simulink model "sm_quadcopter"  (R2022a)
settings: Solver=ode23  StartTime=0.0  StopTime=25  FixedStep=Ts  MaxStep=0.001  RelTol=1e-3  AbsTol=1e-3
model workspace (MATLAB code in the model file):
  | load('xy_data_membrane.mat');
undefined symbols (not defined in the file or in its folder): infPlane, kd_altitude, kd_attitude, kd_position, ki_altitude, ki_attitude, kp_altitude, kp_attitude, kp_position, propeller, targetX, targetY, targetZ, timespot, waypoints, X, x0, xrot, Y, y0, yrot, Z, z0, zrot
libraries: sm_lib x101, fl_lib x40, nesl_utility x36, slpidlib x4
(part 4 of 4)

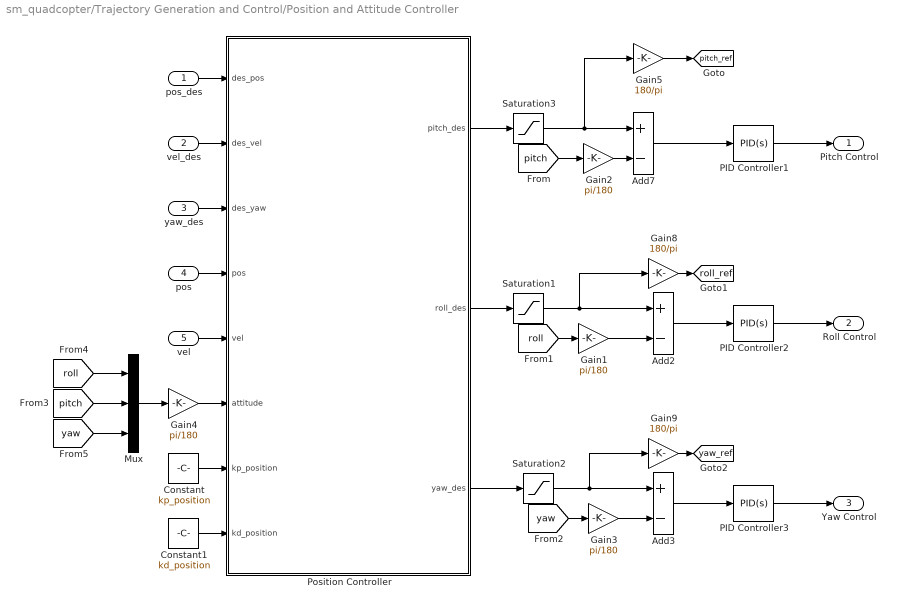
== system sm_quadcopter/Trajectory Generation and Control/Position and Attitude Controller ==
  pos_des : Inport
  vel_des : Inport  Port=2
  yaw_des : Inport  Port=3
  pos : Inport  Port=4
  vel : Inport  Port=5
  Add2 : Sum  Inputs=+-
  Add3 : Sum  Inputs=+-
  Add7 : Sum  Inputs=+-
  Constant : Constant  Value=kp_position
  Constant1 : Constant  Value=kd_position
  Gain{1..4} (4 alike) : Gain  Gain=pi/180
  Gain5 : Gain  Gain=180/pi
  Gain8 : Gain  Gain=180/pi
  Gain9 : Gain  Gain=180/pi
  Mux : Mux  Inputs=3
  PID Controller1 : slpidlib/PID Controller  Controller=PID  Form=Parallel  TimeDomain=Continuous-time  UseExternalTs=off  SampleTime=-1  IntegratorMethod=Forward Euler  FilterMethod=Forward Euler  ControllerParametersSource=internal  P=kp_attitude  I=ki_attitude  UseKiTs=off  D=kd_attitude  N=100  UseFilter=on  TunerSelectOption=Transfer Function Based (PID Tuner App)  InitialConditionSource=internal  InitialConditionForIntegrator=0  InitialConditionForFilter=0  DifferentiatorICPrevScaledInput=0  ExternalReset=none  TrackingMode=off  Kt=1  LimitOutput=on  SatLimitsSource=internal  UpperSaturationLimit=50  LowerSaturationLimit=-50  LinearizeAsGain=on  AntiWindupMode=none  Kb=1  POutMin=[]  POutMax=[]  IOutMin=[]  IOutMax=[]  DOutMin=[]  DOutMax=[]  NOutMin=[]  NOutMax=[]  SumOutMin=[]  SumOutMax=[]  SaturationOutMin=[]  SaturationOutMax=[]  PParamMin=[]  PParamMax=[]  IParamMin=[]  IParamMax=[]  DParamMin=[]  DParamMax=[]  NParamMin=[]  NParamMax=[]  KbParamMin=[]  KbParamMax=[]  KtParamMin=[]  KtParamMax=[]  KbOutMin=[]  KbOutMax=[]  KtOutMin=[]  KtOutMax=[]  IntegratorOutMin=[]  IntegratorOutMax=[]  FilterOutMin=[]  FilterOutMax=[]  SumI1OutMin=[]  SumI1OutMax=[]  SumI2OutMin=[]  SumI2OutMax=[]  SumI3OutMin=[]  SumI3OutMax=[]  SumI4OutMin=[]  SumI4OutMax=[]  SumDOutMin=[]  SumDOutMax=[]  DifferentiatorOutMin=[]  DifferentiatorOutMax=[]  FilterDiffOutCoefMin=[]  FilterDiffOutCoefMax=[]  ReciprocalOutMin=[]  ReciprocalOutMax=[]  SumDenOutMin=[]  SumDenOutMax=[]  SumNumOutMin=[]  SumNumOutMax=[]  DivideOutMin=[]  DivideOutMax=[]  UdiffTsProdOutMin=[]  UdiffTsProdOutMax=[]  NTsProdOutMin=[]  NTsProdOutMax=[]  UintegralTsProdOutMin=[]  UintegralTsProdOutMax=[]  UngainTsProdOutMin=[]  UngainTsProdOutMax=[]  IntegratorContinuousStateAttributes=''  IntegratorStateMustResolveToSignalObject=off  IntegratorRTWStateStorageClass=Auto  FilterContinuousStateAttributes=''  FilterStateMustResolveToSignalObject=off  FilterRTWStateStorageClass=Auto  ParallelPVariant=InternalParameters  IdealPVariant=Disabled  IVariant=InternalParameters  DVariant=InternalParameters  IntegratorVariant=Continuous  SatVariant=Enabled  AWVariant=Passthrough  PCopyVariant=Disabled  TRVariant=Disabled  FdbkBlocksVariant=Forward  IdealPFdbkVariant=Disabled  SatFdbkVariant=Disabled  DerivativeFilterVariant=ContFilter  NVariant=InternalParameters  NCopyVariant=Disabled  FilterICVariant=InternalICsFilter  IntegratorICVariant=InternalICs  ExternalResetVariant=Disabled  TRSumVariant=Passthrough  SumFdbkVariant=Disabled  SumVariant=Sum_PID  TsampFilterVariant=InternalTs  TsampNgainVariant=Passthrough  TsampIntegralVariant=Passthrough  ExternalSaturationOutDataTypeStr=Inherit: Same as second input  aMode=0
  PID Controller2 : slpidlib/PID Controller  Controller=PID  Form=Parallel  TimeDomain=Continuous-time  UseExternalTs=off  SampleTime=-1  IntegratorMethod=Forward Euler  FilterMethod=Forward Euler  ControllerParametersSource=internal  P=kp_attitude  I=ki_attitude  UseKiTs=off  D=kd_attitude  N=100  UseFilter=on  TunerSelectOption=Transfer Function Based (PID Tuner App)  InitialConditionSource=internal  InitialConditionForIntegrator=0  InitialConditionForFilter=0  DifferentiatorICPrevScaledInput=0  ExternalReset=none  TrackingMode=off  Kt=1  LimitOutput=on  SatLimitsSource=internal  UpperSaturationLimit=50  LowerSaturationLimit=-50  LinearizeAsGain=on  AntiWindupMode=none  Kb=1  POutMin=[]  POutMax=[]  IOutMin=[]  IOutMax=[]  DOutMin=[]  DOutMax=[]  NOutMin=[]  NOutMax=[]  SumOutMin=[]  SumOutMax=[]  SaturationOutMin=[]  SaturationOutMax=[]  PParamMin=[]  PParamMax=[]  IParamMin=[]  IParamMax=[]  DParamMin=[]  DParamMax=[]  NParamMin=[]  NParamMax=[]  KbParamMin=[]  KbParamMax=[]  KtParamMin=[]  KtParamMax=[]  KbOutMin=[]  KbOutMax=[]  KtOutMin=[]  KtOutMax=[]  IntegratorOutMin=[]  IntegratorOutMax=[]  FilterOutMin=[]  FilterOutMax=[]  SumI1OutMin=[]  SumI1OutMax=[]  SumI2OutMin=[]  SumI2OutMax=[]  SumI3OutMin=[]  SumI3OutMax=[]  SumI4OutMin=[]  SumI4OutMax=[]  SumDOutMin=[]  SumDOutMax=[]  DifferentiatorOutMin=[]  DifferentiatorOutMax=[]  FilterDiffOutCoefMin=[]  FilterDiffOutCoefMax=[]  ReciprocalOutMin=[]  ReciprocalOutMax=[]  SumDenOutMin=[]  SumDenOutMax=[]  SumNumOutMin=[]  SumNumOutMax=[]  DivideOutMin=[]  DivideOutMax=[]  UdiffTsProdOutMin=[]  UdiffTsProdOutMax=[]  NTsProdOutMin=[]  NTsProdOutMax=[]  UintegralTsProdOutMin=[]  UintegralTsProdOutMax=[]  UngainTsProdOutMin=[]  UngainTsProdOutMax=[]  IntegratorContinuousStateAttributes=''  IntegratorStateMustResolveToSignalObject=off  IntegratorRTWStateStorageClass=Auto  FilterContinuousStateAttributes=''  FilterStateMustResolveToSignalObject=off  FilterRTWStateStorageClass=Auto  ParallelPVariant=InternalParameters  IdealPVariant=Disabled  IVariant=InternalParameters  DVariant=InternalParameters  IntegratorVariant=Continuous  SatVariant=Enabled  AWVariant=Passthrough  PCopyVariant=Disabled  TRVariant=Disabled  FdbkBlocksVariant=Forward  IdealPFdbkVariant=Disabled  SatFdbkVariant=Disabled  DerivativeFilterVariant=ContFilter  NVariant=InternalParameters  NCopyVariant=Disabled  FilterICVariant=InternalICsFilter  IntegratorICVariant=InternalICs  ExternalResetVariant=Disabled  TRSumVariant=Passthrough  SumFdbkVariant=Disabled  SumVariant=Sum_PID  TsampFilterVariant=InternalTs  TsampNgainVariant=Passthrough  TsampIntegralVariant=Passthrough  ExternalSaturationOutDataTypeStr=Inherit: Same as second input  aMode=0
  PID Controller3 : slpidlib/PID Controller  Controller=PID  Form=Parallel  TimeDomain=Continuous-time  UseExternalTs=off  SampleTime=-1  IntegratorMethod=Forward Euler  FilterMethod=Forward Euler  ControllerParametersSource=internal  P=kp_attitude  I=ki_attitude  UseKiTs=off  D=kd_attitude  N=100  UseFilter=on  TunerSelectOption=Transfer Function Based (PID Tuner App)  InitialConditionSource=internal  InitialConditionForIntegrator=0  InitialConditionForFilter=0  DifferentiatorICPrevScaledInput=0  ExternalReset=none  TrackingMode=off  Kt=1  LimitOutput=on  SatLimitsSource=internal  UpperSaturationLimit=50  LowerSaturationLimit=-50  LinearizeAsGain=on  AntiWindupMode=none  Kb=1  POutMin=[]  POutMax=[]  IOutMin=[]  IOutMax=[]  DOutMin=[]  DOutMax=[]  NOutMin=[]  NOutMax=[]  SumOutMin=[]  SumOutMax=[]  SaturationOutMin=[]  SaturationOutMax=[]  PParamMin=[]  PParamMax=[]  IParamMin=[]  IParamMax=[]  DParamMin=[]  DParamMax=[]  NParamMin=[]  NParamMax=[]  KbParamMin=[]  KbParamMax=[]  KtParamMin=[]  KtParamMax=[]  KbOutMin=[]  KbOutMax=[]  KtOutMin=[]  KtOutMax=[]  IntegratorOutMin=[]  IntegratorOutMax=[]  FilterOutMin=[]  FilterOutMax=[]  SumI1OutMin=[]  SumI1OutMax=[]  SumI2OutMin=[]  SumI2OutMax=[]  SumI3OutMin=[]  SumI3OutMax=[]  SumI4OutMin=[]  SumI4OutMax=[]  SumDOutMin=[]  SumDOutMax=[]  DifferentiatorOutMin=[]  DifferentiatorOutMax=[]  FilterDiffOutCoefMin=[]  FilterDiffOutCoefMax=[]  ReciprocalOutMin=[]  ReciprocalOutMax=[]  SumDenOutMin=[]  SumDenOutMax=[]  SumNumOutMin=[]  SumNumOutMax=[]  DivideOutMin=[]  DivideOutMax=[]  UdiffTsProdOutMin=[]  UdiffTsProdOutMax=[]  NTsProdOutMin=[]  NTsProdOutMax=[]  UintegralTsProdOutMin=[]  UintegralTsProdOutMax=[]  UngainTsProdOutMin=[]  UngainTsProdOutMax=[]  IntegratorContinuousStateAttributes=''  IntegratorStateMustResolveToSignalObject=off  IntegratorRTWStateStorageClass=Auto  FilterContinuousStateAttributes=''  FilterStateMustResolveToSignalObject=off  FilterRTWStateStorageClass=Auto  ParallelPVariant=InternalParameters  IdealPVariant=Disabled  IVariant=InternalParameters  DVariant=InternalParameters  IntegratorVariant=Continuous  SatVariant=Enabled  AWVariant=Passthrough  PCopyVariant=Disabled  TRVariant=Disabled  FdbkBlocksVariant=Forward  IdealPFdbkVariant=Disabled  SatFdbkVariant=Disabled  DerivativeFilterVariant=ContFilter  NVariant=InternalParameters  NCopyVariant=Disabled  FilterICVariant=InternalICsFilter  IntegratorICVariant=InternalICs  ExternalResetVariant=Disabled  TRSumVariant=Passthrough  SumFdbkVariant=Disabled  SumVariant=Sum_PID  TsampFilterVariant=InternalTs  TsampNgainVariant=Passthrough  TsampIntegralVariant=Passthrough  ExternalSaturationOutDataTypeStr=Inherit: Same as second input  aMode=0
  Position Controller : MATLAB Function  TreatAsAtomicUnit=on
  Saturation1 : Saturate  UpperLimit=pi/3  LowerLimit=-pi/3
  Saturation2 : Saturate  UpperLimit=pi/3  LowerLimit=-pi/3
  Saturation3 : Saturate  UpperLimit=pi/3  LowerLimit=-pi/3
  Pitch Control : Outport
  Roll Control : Outport  Port=2
  Yaw Control : Outport  Port=3
  tag scope: pitch_ref=global, roll_ref=global, yaw_ref=global
  wires:
  pos/1 -> Position Controller/4(pos)
  pos_des/1 -> Position Controller/1(des_pos)
  Position Controller/2(roll_des) -> Saturation1/1
  Saturation2/1 -> Gain9/1, Add3/1
  Position Controller/3(yaw_des) -> Saturation2/1
  yaw_des/1 -> Position Controller/3(des_yaw)
  vel/1 -> Position Controller/5(vel)
  [yaw] -> Gain3/1
  [roll] -> Gain1/1
  [pitch] -> Gain2/1
  vel_des/1 -> Position Controller/2(des_vel)
  Saturation1/1 -> Gain8/1, Add2/1
  Saturation3/1 -> Add7/1, Gain5/1
  Position Controller/1(pitch_des) -> Saturation3/1
  Mux/1 -> Gain4/1
  [roll] -> Mux/1
  [pitch] -> Mux/2
  [yaw] -> Mux/3
  Gain4/1 -> Position Controller/6(attitude)
  Gain1/1 -> Add2/2
  Gain3/1 -> Add3/2
  Gain5/1 -> [pitch_ref]
  Gain8/1 -> [roll_ref]
  Gain9/1 -> [yaw_ref]
  Gain2/1 -> Add7/2
  Add7/1 -> PID Controller1/1
  PID Controller1/1 -> Pitch Control/1
  Add2/1 -> PID Controller2/1
  PID Controller2/1 -> Roll Control/1
  Add3/1 -> PID Controller3/1
  PID Controller3/1 -> Yaw Control/1
  Constant/1 -> Position Controller/7(kp_position)
  Constant1/1 -> Position Controller/8(kd_position)

== system sm_quadcopter/Package Delivery Quadcopter/Motor Propeller 1/Propeller Thrust Calculator ==
  Air Density : fl_lib/Physical Signals/Sources/PS Constant  constant=1.225 kg/m^3
      settings: SourceProductBaseCode=PW,SS,VE
  PS Gain : fl_lib/Physical Signals/Functions/PS Gain  gain=1/60
      settings: SourceProductBaseCode=PW,SS,VE
  PS Math Function : fl_lib/Physical Signals/Functions/PS Math Function  fcn_choice=foundation.enum.math_function.pow  v=4
      settings: SourceProductBaseCode=PW,SS,VE
  PS Math Function1 : fl_lib/Physical Signals/Functions/PS Math Function  fcn_choice=foundation.enum.math_function.square  v=2
      settings: SourceProductBaseCode=PW,SS,VE
  PS Product : fl_lib/Physical Signals/Functions/PS Product
      settings: SourceProductBaseCode=PW,SS,VE
  PS Product1 : fl_lib/Physical Signals/Functions/PS Product
      settings: SourceProductBaseCode=PW,SS,VE
  PS Product2 : fl_lib/Physical Signals/Functions/PS Product
      settings: SourceProductBaseCode=PW,SS,VE
  Propeller Diameter : fl_lib/Physical Signals/Sources/PS Constant  constant=propeller.diameter m
      settings: SourceProductBaseCode=PW,SS,VE
  Ct : PMIOPort  Side=Left
  Propeller Speed : PMIOPort  Port=2  Side=Left
  Thrust : PMIOPort  Port=3  Side=Right
  connections:
  PS Math Function/LConn1 -- Propeller Diameter/RConn1
  PS Math Function1/RConn1 -- PS Product1/LConn1
  Air Density/RConn1 -- PS Product1/LConn2
  PS Product1/RConn1 -- PS Product2/LConn2
  PS Gain/RConn1 -- PS Math Function1/LConn1
  PS Math Function/RConn1 -- PS Product/LConn2
  PS Product/RConn1 -- PS Product2/LConn1
  Propeller Speed/RConn1 -- PS Gain/LConn1
  Thrust/RConn1 -- PS Product2/RConn1
  PS Product/LConn1 -- Ct/RConn1

== system sm_quadcopter/Package Delivery Quadcopter/Motor Propeller 1/Thrust Coefficient Calculator ==
  m/s : Inport
  Add : Sum  Inputs=+++
  Constant : Constant  Value=0.1072
  Gain1 : Gain  Gain=-0.008716
  Gain4 : Gain  Gain=-0.001589
  Math Function : Math  Operator=square
  Simulink-PS Converter : nesl_utility/Simulink-PS Converter  PhysicalDomain=network_engine_domain  SubClassName=ps_input  LeftPortType=input  RightPortType=output  PseudoPeriodic=off  Frequencies=[]  NoiseDistribution=none  NoiseParameters=[]  Unit=1/(rev)^2  AffineConversion=off  FilteringAndDerivatives=provide  SimscapeFilterOrder=1  InputFilterTimeConstant=0.001  UdotUserProvided=0
      settings: SourceProductBaseCode=SS,PW,VE
  Ct : PMIOPort  Side=Right
  wires:
  Constant/1 -> Add/3
  Gain4/1 -> Add/1
  Add/1 -> Simulink-PS Converter/1
  m/s/1 -> Gain1/1, Math Function/1
  Math Function/1 -> Gain4/1
  Gain1/1 -> Add/2
  connections:
  Simulink-PS Converter/RConn1 -- Ct/RConn1

== system sm_quadcopter/Package Delivery Quadcopter/Motor Propeller 2/Propeller Thrust Calculator ==
  Air Density : fl_lib/Physical Signals/Sources/PS Constant  constant=1.225 kg/m^3
      settings: SourceProductBaseCode=PW,SS,VE
  PS Gain : fl_lib/Physical Signals/Functions/PS Gain  gain=1/60
      settings: SourceProductBaseCode=PW,SS,VE
  PS Math Function : fl_lib/Physical Signals/Functions/PS Math Function  fcn_choice=foundation.enum.math_function.pow  v=4
      settings: SourceProductBaseCode=PW,SS,VE
  PS Math Function1 : fl_lib/Physical Signals/Functions/PS Math Function  fcn_choice=foundation.enum.math_function.square  v=2
      settings: SourceProductBaseCode=PW,SS,VE
  PS Product : fl_lib/Physical Signals/Functions/PS Product
      settings: SourceProductBaseCode=PW,SS,VE
  PS Product1 : fl_lib/Physical Signals/Functions/PS Product
      settings: SourceProductBaseCode=PW,SS,VE
  PS Product2 : fl_lib/Physical Signals/Functions/PS Product
      settings: SourceProductBaseCode=PW,SS,VE
  Propeller Diameter : fl_lib/Physical Signals/Sources/PS Constant  constant=propeller.diameter m
      settings: SourceProductBaseCode=PW,SS,VE
  Ct : PMIOPort  Side=Left
  Propeller Speed : PMIOPort  Port=2  Side=Left
  Thrust : PMIOPort  Port=3  Side=Right
  connections:
  PS Math Function/LConn1 -- Propeller Diameter/RConn1
  PS Math Function1/RConn1 -- PS Product1/LConn1
  Air Density/RConn1 -- PS Product1/LConn2
  PS Product1/RConn1 -- PS Product2/LConn2
  PS Gain/RConn1 -- PS Math Function1/LConn1
  PS Math Function/RConn1 -- PS Product/LConn2
  PS Product/RConn1 -- PS Product2/LConn1
  Propeller Speed/RConn1 -- PS Gain/LConn1
  Thrust/RConn1 -- PS Product2/RConn1
  PS Product/LConn1 -- Ct/RConn1

== system sm_quadcopter/Package Delivery Quadcopter/Motor Propeller 2/Thrust Coefficient Calculator ==
  m/s : Inport
  Add : Sum  Inputs=+++
  Constant : Constant  Value=0.1072
  Gain1 : Gain  Gain=-0.008716
  Gain4 : Gain  Gain=-0.001589
  Math Function : Math  Operator=square
  Simulink-PS Converter : nesl_utility/Simulink-PS Converter  PhysicalDomain=network_engine_domain  SubClassName=ps_input  LeftPortType=input  RightPortType=output  PseudoPeriodic=off  Frequencies=[]  NoiseDistribution=none  NoiseParameters=[]  Unit=1/(rev^2)  AffineConversion=off  FilteringAndDerivatives=provide  SimscapeFilterOrder=1  InputFilterTimeConstant=0.001  UdotUserProvided=0
      settings: SourceProductBaseCode=SS,PW,VE
  Ct : PMIOPort  Side=Right
  wires:
  Math Function/1 -> Gain4/1
  m/s/1 -> Gain1/1, Math Function/1
  Add/1 -> Simulink-PS Converter/1
  Gain4/1 -> Add/1
  Gain1/1 -> Add/2
  Constant/1 -> Add/3
  connections:
  Simulink-PS Converter/RConn1 -- Ct/RConn1

== system sm_quadcopter/Package Delivery Quadcopter/Motor Propeller 3 /Propeller Thrust Calculator ==
  Air Density : fl_lib/Physical Signals/Sources/PS Constant  constant=1.225 kg/m^3
      settings: SourceProductBaseCode=PW,SS,VE
  PS Gain : fl_lib/Physical Signals/Functions/PS Gain  gain=1/60
      settings: SourceProductBaseCode=PW,SS,VE
  PS Math Function : fl_lib/Physical Signals/Functions/PS Math Function  fcn_choice=foundation.enum.math_function.pow  v=4
      settings: SourceProductBaseCode=PW,SS,VE
  PS Math Function1 : fl_lib/Physical Signals/Functions/PS Math Function  fcn_choice=foundation.enum.math_function.square  v=2
      settings: SourceProductBaseCode=PW,SS,VE
  PS Product : fl_lib/Physical Signals/Functions/PS Product
      settings: SourceProductBaseCode=PW,SS,VE
  PS Product1 : fl_lib/Physical Signals/Functions/PS Product
      settings: SourceProductBaseCode=PW,SS,VE
  PS Product2 : fl_lib/Physical Signals/Functions/PS Product
      settings: SourceProductBaseCode=PW,SS,VE
  Propeller Diameter : fl_lib/Physical Signals/Sources/PS Constant  constant=propeller.diameter m
      settings: SourceProductBaseCode=PW,SS,VE
  Ct : PMIOPort  Side=Left
  Propeller Speed : PMIOPort  Port=2  Side=Left
  Thrust : PMIOPort  Port=3  Side=Right
  connections:
  PS Math Function/LConn1 -- Propeller Diameter/RConn1
  PS Math Function1/RConn1 -- PS Product1/LConn1
  Air Density/RConn1 -- PS Product1/LConn2
  PS Product1/RConn1 -- PS Product2/LConn2
  PS Math Function/RConn1 -- PS Product/LConn2
  PS Product/RConn1 -- PS Product2/LConn1
  PS Math Function1/LConn1 -- PS Gain/RConn1
  Propeller Speed/RConn1 -- PS Gain/LConn1
  Thrust/RConn1 -- PS Product2/RConn1
  PS Product/LConn1 -- Ct/RConn1

== system sm_quadcopter/Package Delivery Quadcopter/Motor Propeller 3 /Thrust Coefficient Calculator ==
  m/s : Inport
  Add : Sum  Inputs=+++
  Constant : Constant  Value=0.1072
  Gain1 : Gain  Gain=-0.008716
  Gain4 : Gain  Gain=-0.001589
  Math Function : Math  Operator=square
  Simulink-PS Converter : nesl_utility/Simulink-PS Converter  PhysicalDomain=network_engine_domain  SubClassName=ps_input  LeftPortType=input  RightPortType=output  PseudoPeriodic=off  Frequencies=[]  NoiseDistribution=none  NoiseParameters=[]  Unit=1/(rev)^2  AffineConversion=off  FilteringAndDerivatives=provide  SimscapeFilterOrder=1  InputFilterTimeConstant=0.001  UdotUserProvided=0
      settings: SourceProductBaseCode=SS,PW,VE
  Ct : PMIOPort  Side=Right
  wires:
  Constant/1 -> Add/3
  Gain4/1 -> Add/1
  Add/1 -> Simulink-PS Converter/1
  m/s/1 -> Gain1/1, Math Function/1
  Math Function/1 -> Gain4/1
  Gain1/1 -> Add/2
  connections:
  Simulink-PS Converter/RConn1 -- Ct/RConn1

== system sm_quadcopter/Package Delivery Quadcopter/Motor Propeller 4/Propeller Thrust Calculator ==
  Air Density : fl_lib/Physical Signals/Sources/PS Constant  constant=1.225 kg/m^3
      settings: SourceProductBaseCode=PW,SS,VE
  PS Gain : fl_lib/Physical Signals/Functions/PS Gain  gain=1/60
      settings: SourceProductBaseCode=PW,SS,VE
  PS Math Function : fl_lib/Physical Signals/Functions/PS Math Function  fcn_choice=foundation.enum.math_function.pow  v=4
      settings: SourceProductBaseCode=PW,SS,VE
  PS Math Function1 : fl_lib/Physical Signals/Functions/PS Math Function  fcn_choice=foundation.enum.math_function.square  v=2
      settings: SourceProductBaseCode=PW,SS,VE
  PS Product : fl_lib/Physical Signals/Functions/PS Product
      settings: SourceProductBaseCode=PW,SS,VE
  PS Product1 : fl_lib/Physical Signals/Functions/PS Product
      settings: SourceProductBaseCode=PW,SS,VE
  PS Product2 : fl_lib/Physical Signals/Functions/PS Product
      settings: SourceProductBaseCode=PW,SS,VE
  Propeller Diameter : fl_lib/Physical Signals/Sources/PS Constant  constant=propeller.diameter m
      settings: SourceProductBaseCode=PW,SS,VE
  Ct : PMIOPort  Side=Left
  Propeller Speed : PMIOPort  Port=2  Side=Left
  Thrust : PMIOPort  Port=3  Side=Right
  connections:
  PS Math Function/LConn1 -- Propeller Diameter/RConn1
  PS Math Function1/RConn1 -- PS Product1/LConn1
  Air Density/RConn1 -- PS Product1/LConn2
  PS Product1/RConn1 -- PS Product2/LConn2
  PS Gain/RConn1 -- PS Math Function1/LConn1
  PS Math Function/RConn1 -- PS Product/LConn2
  PS Product/RConn1 -- PS Product2/LConn1
  Propeller Speed/RConn1 -- PS Gain/LConn1
  Thrust/RConn1 -- PS Product2/RConn1
  PS Product/LConn1 -- Ct/RConn1

== system sm_quadcopter/Package Delivery Quadcopter/Motor Propeller 4/Thrust Coefficient Calculator ==
  m/s : Inport
  Add : Sum  Inputs=+++
  Constant : Constant  Value=0.1072
  Gain1 : Gain  Gain=-0.008716
  Gain4 : Gain  Gain=-0.001589
  Math Function : Math  Operator=square
  Simulink-PS Converter : nesl_utility/Simulink-PS Converter  PhysicalDomain=network_engine_domain  SubClassName=ps_input  LeftPortType=input  RightPortType=output  PseudoPeriodic=off  Frequencies=[]  NoiseDistribution=none  NoiseParameters=[]  Unit=1/(rev)^2  AffineConversion=off  FilteringAndDerivatives=provide  SimscapeFilterOrder=1  InputFilterTimeConstant=0.001  UdotUserProvided=0
      settings: SourceProductBaseCode=SS,PW,VE
  Ct : PMIOPort  Side=Right
  wires:
  Constant/1 -> Add/3
  Gain4/1 -> Add/1
  Add/1 -> Simulink-PS Converter/1
  m/s/1 -> Gain1/1, Math Function/1
  Math Function/1 -> Gain4/1
  Gain1/1 -> Add/2
  connections:
  Simulink-PS Converter/RConn1 -- Ct/RConn1

== system sm_quadcopter/Package Delivery Quadcopter/Package/Subsystem ==
  Spatial Contact Force : sm_lib/Forces and Torques/Spatial Contact Force  SenseContactBaseRotation=off  SenseContactBaseTranslation=off  CoefficientOfDynamicFriction=0.3  CoefficientOfStaticFriction=0.5  NormalDamping=pkgGrndDamp  NormalDampingUnits=N/(m/s)  SenseContactSignal=off  NormalStiffness=pkgGrndStiff  NormalStiffnessUnits=N/m  FrictionalCriticalVelocity=1e-2  FrictionalCriticalVelocityUnits=m/s  ZeroCrossDetectContactStartAndEnd=off  SenseContactFollowerRotation=off  SenseContactFollowerTranslation=off  FrictionType=SmoothStickSlip  SenseFrictionalForceMagnitude=off  SenseNormalForceMagnitude=off  NormalForceType=SmoothSpringDamper  SenseNormalVelocity=off  SenseSeparationDistance=off  SenseTangentialVelocity=off  NormalTransitionRegionWidth=pkgGrndTransW  NormalTransitionRegionWidthUnits=m
  Spherical Solid : sm_lib/Body Elements/Spherical Solid  GraphicAmbientColor=[0.15 0.15 0.15 1.0]  BasedOnType=Density  CenterOfMass=[0 0 0]  CenterOfMassUnits=m  GraphicDiffuseColor=[0.5 0.5 0.5]  Density=1  DensityUnits=kg/m^3  DoExposeReferenceFrame=on  GraphicEmissiveColor=[0.0 0.0 0.0 1.0]  ExportEntireGeometry=on  SerializedExposedGeometries=<ExposedGeometries><ExposedGeometry><RawGeometryId>entire</RawGeometryId><ExposedGeometryId>G</ExposedGeometryId></ExposedGeometry></ExposedGeometries>  SerializedFrames=<Frames/>  MarkerShape=Sphere  MarkerSize=10  GraphicType=FromGeometry  InertiaType=CalculateFromGeometry  Mass=1  MassUnits=kg  MomentsOfInertia=[1 1 1]  MomentsOfInertiaUnits=kg*m^2  GraphicOpacity=1.0  ProductsOfInertia=[0 0 0]  ProductsOfInertiaUnits=kg*m^2  GraphicShininess=75  GraphicSpecularColor=[0.5 0.5 0.5 1.0]  SphereRadius=0.0025  SphereRadiusUnits=m  GraphicVisPropType=SimpleVisualProperties
  R : PMIOPort  Side=Right
  G : PMIOPort  Port=2  Side=Left
  connections:
  Spatial Contact Force/LConn1 -- Spherical Solid/LConn1
  Spherical Solid/RConn1 -- R/RConn1
  Spatial Contact Force/RConn1 -- G/RConn1

== system sm_quadcopter/Package Delivery Quadcopter/Package/Subsystem1 ==
  Spatial Contact Force : sm_lib/Forces and Torques/Spatial Contact Force  SenseContactBaseRotation=off  SenseContactBaseTranslation=off  CoefficientOfDynamicFriction=0.3  CoefficientOfStaticFriction=0.5  NormalDamping=pkgGrndDamp  NormalDampingUnits=N/(m/s)  SenseContactSignal=off  NormalStiffness=pkgGrndStiff  NormalStiffnessUnits=N/m  FrictionalCriticalVelocity=1e-2  FrictionalCriticalVelocityUnits=m/s  ZeroCrossDetectContactStartAndEnd=off  SenseContactFollowerRotation=off  SenseContactFollowerTranslation=off  FrictionType=SmoothStickSlip  SenseFrictionalForceMagnitude=off  SenseNormalForceMagnitude=off  NormalForceType=SmoothSpringDamper  SenseNormalVelocity=off  SenseSeparationDistance=off  SenseTangentialVelocity=off  NormalTransitionRegionWidth=pkgGrndTransW  NormalTransitionRegionWidthUnits=m
  Spherical Solid : sm_lib/Body Elements/Spherical Solid  GraphicAmbientColor=[0.15 0.15 0.15 1.0]  BasedOnType=Density  CenterOfMass=[0 0 0]  CenterOfMassUnits=m  GraphicDiffuseColor=[0.5 0.5 0.5]  Density=1  DensityUnits=kg/m^3  DoExposeReferenceFrame=on  GraphicEmissiveColor=[0.0 0.0 0.0 1.0]  ExportEntireGeometry=on  SerializedExposedGeometries=<ExposedGeometries><ExposedGeometry><RawGeometryId>entire</RawGeometryId><ExposedGeometryId>G</ExposedGeometryId></ExposedGeometry></ExposedGeometries>  SerializedFrames=<Frames/>  MarkerShape=Sphere  MarkerSize=10  GraphicType=FromGeometry  InertiaType=CalculateFromGeometry  Mass=1  MassUnits=kg  MomentsOfInertia=[1 1 1]  MomentsOfInertiaUnits=kg*m^2  GraphicOpacity=1.0  ProductsOfInertia=[0 0 0]  ProductsOfInertiaUnits=kg*m^2  GraphicShininess=75  GraphicSpecularColor=[0.5 0.5 0.5 1.0]  SphereRadius=0.0025  SphereRadiusUnits=m  GraphicVisPropType=SimpleVisualProperties
  R : PMIOPort  Side=Right
  G : PMIOPort  Port=2  Side=Left
  connections:
  Spatial Contact Force/RConn1 -- G/RConn1
  Spherical Solid/RConn1 -- R/RConn1
  Spatial Contact Force/LConn1 -- Spherical Solid/LConn1

== system sm_quadcopter/Package Delivery Quadcopter/Package/Subsystem2 ==
  Spatial Contact Force : sm_lib/Forces and Torques/Spatial Contact Force  SenseContactBaseRotation=off  SenseContactBaseTranslation=off  CoefficientOfDynamicFriction=0.3  CoefficientOfStaticFriction=0.5  NormalDamping=pkgGrndDamp  NormalDampingUnits=N/(m/s)  SenseContactSignal=off  NormalStiffness=pkgGrndStiff  NormalStiffnessUnits=N/m  FrictionalCriticalVelocity=1e-2  FrictionalCriticalVelocityUnits=m/s  ZeroCrossDetectContactStartAndEnd=off  SenseContactFollowerRotation=off  SenseContactFollowerTranslation=off  FrictionType=SmoothStickSlip  SenseFrictionalForceMagnitude=off  SenseNormalForceMagnitude=off  NormalForceType=SmoothSpringDamper  SenseNormalVelocity=off  SenseSeparationDistance=off  SenseTangentialVelocity=off  NormalTransitionRegionWidth=pkgGrndTransW  NormalTransitionRegionWidthUnits=m
  Spherical Solid : sm_lib/Body Elements/Spherical Solid  GraphicAmbientColor=[0.15 0.15 0.15 1.0]  BasedOnType=Density  CenterOfMass=[0 0 0]  CenterOfMassUnits=m  GraphicDiffuseColor=[0.5 0.5 0.5]  Density=1  DensityUnits=kg/m^3  DoExposeReferenceFrame=on  GraphicEmissiveColor=[0.0 0.0 0.0 1.0]  ExportEntireGeometry=on  SerializedExposedGeometries=<ExposedGeometries><ExposedGeometry><RawGeometryId>entire</RawGeometryId><ExposedGeometryId>G</ExposedGeometryId></ExposedGeometry></ExposedGeometries>  SerializedFrames=<Frames/>  MarkerShape=Sphere  MarkerSize=10  GraphicType=FromGeometry  InertiaType=CalculateFromGeometry  Mass=1  MassUnits=kg  MomentsOfInertia=[1 1 1]  MomentsOfInertiaUnits=kg*m^2  GraphicOpacity=1.0  ProductsOfInertia=[0 0 0]  ProductsOfInertiaUnits=kg*m^2  GraphicShininess=75  GraphicSpecularColor=[0.5 0.5 0.5 1.0]  SphereRadius=0.0025  SphereRadiusUnits=m  GraphicVisPropType=SimpleVisualProperties
  R : PMIOPort  Side=Right
  G : PMIOPort  Port=2  Side=Left
  connections:
  Spatial Contact Force/LConn1 -- Spherical Solid/LConn1
  Spherical Solid/RConn1 -- R/RConn1
  Spatial Contact Force/RConn1 -- G/RConn1

== system sm_quadcopter/Package Delivery Quadcopter/Package/Subsystem3 ==
  Spatial Contact Force : sm_lib/Forces and Torques/Spatial Contact Force  SenseContactBaseRotation=off  SenseContactBaseTranslation=off  CoefficientOfDynamicFriction=0.3  CoefficientOfStaticFriction=0.5  NormalDamping=pkgGrndDamp  NormalDampingUnits=N/(m/s)  SenseContactSignal=off  NormalStiffness=pkgGrndStiff  NormalStiffnessUnits=N/m  FrictionalCriticalVelocity=1e-2  FrictionalCriticalVelocityUnits=m/s  ZeroCrossDetectContactStartAndEnd=off  SenseContactFollowerRotation=off  SenseContactFollowerTranslation=off  FrictionType=SmoothStickSlip  SenseFrictionalForceMagnitude=off  SenseNormalForceMagnitude=off  NormalForceType=SmoothSpringDamper  SenseNormalVelocity=off  SenseSeparationDistance=off  SenseTangentialVelocity=off  NormalTransitionRegionWidth=pkgGrndTransW  NormalTransitionRegionWidthUnits=m
  Spherical Solid : sm_lib/Body Elements/Spherical Solid  GraphicAmbientColor=[0.15 0.15 0.15 1.0]  BasedOnType=Density  CenterOfMass=[0 0 0]  CenterOfMassUnits=m  GraphicDiffuseColor=[0.5 0.5 0.5]  Density=1  DensityUnits=kg/m^3  DoExposeReferenceFrame=on  GraphicEmissiveColor=[0.0 0.0 0.0 1.0]  ExportEntireGeometry=on  SerializedExposedGeometries=<ExposedGeometries><ExposedGeometry><RawGeometryId>entire</RawGeometryId><ExposedGeometryId>G</ExposedGeometryId></ExposedGeometry></ExposedGeometries>  SerializedFrames=<Frames/>  MarkerShape=Sphere  MarkerSize=10  GraphicType=FromGeometry  InertiaType=CalculateFromGeometry  Mass=1  MassUnits=kg  MomentsOfInertia=[1 1 1]  MomentsOfInertiaUnits=kg*m^2  GraphicOpacity=1.0  ProductsOfInertia=[0 0 0]  ProductsOfInertiaUnits=kg*m^2  GraphicShininess=75  GraphicSpecularColor=[0.5 0.5 0.5 1.0]  SphereRadius=0.0025  SphereRadiusUnits=m  GraphicVisPropType=SimpleVisualProperties
  R : PMIOPort  Side=Right
  G : PMIOPort  Port=2  Side=Left
  connections:
  Spatial Contact Force/RConn1 -- G/RConn1
  Spherical Solid/RConn1 -- R/RConn1
  Spatial Contact Force/LConn1 -- Spherical Solid/LConn1

== system sm_quadcopter/Package Delivery Quadcopter/Package/Subsystem4 ==
  Spatial Contact Force : sm_lib/Forces and Torques/Spatial Contact Force  SenseContactBaseRotation=off  SenseContactBaseTranslation=off  CoefficientOfDynamicFriction=0.3  CoefficientOfStaticFriction=0.5  NormalDamping=pkgGrndDamp  NormalDampingUnits=N/(m/s)  SenseContactSignal=off  NormalStiffness=pkgGrndStiff  NormalStiffnessUnits=N/m  FrictionalCriticalVelocity=1e-2  FrictionalCriticalVelocityUnits=m/s  ZeroCrossDetectContactStartAndEnd=off  SenseContactFollowerRotation=off  SenseContactFollowerTranslation=off  FrictionType=SmoothStickSlip  SenseFrictionalForceMagnitude=off  SenseNormalForceMagnitude=off  NormalForceType=SmoothSpringDamper  SenseNormalVelocity=off  SenseSeparationDistance=off  SenseTangentialVelocity=off  NormalTransitionRegionWidth=pkgGrndTransW  NormalTransitionRegionWidthUnits=m
  Spherical Solid : sm_lib/Body Elements/Spherical Solid  GraphicAmbientColor=[0.15 0.15 0.15 1.0]  BasedOnType=Density  CenterOfMass=[0 0 0]  CenterOfMassUnits=m  GraphicDiffuseColor=[0.5 0.5 0.5]  Density=1  DensityUnits=kg/m^3  DoExposeReferenceFrame=on  GraphicEmissiveColor=[0.0 0.0 0.0 1.0]  ExportEntireGeometry=on  SerializedExposedGeometries=<ExposedGeometries><ExposedGeometry><RawGeometryId>entire</RawGeometryId><ExposedGeometryId>G</ExposedGeometryId></ExposedGeometry></ExposedGeometries>  SerializedFrames=<Frames/>  MarkerShape=Sphere  MarkerSize=10  GraphicType=FromGeometry  InertiaType=CalculateFromGeometry  Mass=1  MassUnits=kg  MomentsOfInertia=[1 1 1]  MomentsOfInertiaUnits=kg*m^2  GraphicOpacity=1.0  ProductsOfInertia=[0 0 0]  ProductsOfInertiaUnits=kg*m^2  GraphicShininess=75  GraphicSpecularColor=[0.5 0.5 0.5 1.0]  SphereRadius=0.0025  SphereRadiusUnits=m  GraphicVisPropType=SimpleVisualProperties
  R : PMIOPort  Side=Right
  G : PMIOPort  Port=2  Side=Left
  connections:
  Spatial Contact Force/LConn1 -- Spherical Solid/LConn1
  Spherical Solid/RConn1 -- R/RConn1
  Spatial Contact Force/RConn1 -- G/RConn1

== system sm_quadcopter/Package Delivery Quadcopter/Package/Subsystem5 ==
  Spatial Contact Force : sm_lib/Forces and Torques/Spatial Contact Force  SenseContactBaseRotation=off  SenseContactBaseTranslation=off  CoefficientOfDynamicFriction=0.3  CoefficientOfStaticFriction=0.5  NormalDamping=pkgGrndDamp  NormalDampingUnits=N/(m/s)  SenseContactSignal=off  NormalStiffness=pkgGrndStiff  NormalStiffnessUnits=N/m  FrictionalCriticalVelocity=1e-2  FrictionalCriticalVelocityUnits=m/s  ZeroCrossDetectContactStartAndEnd=off  SenseContactFollowerRotation=off  SenseContactFollowerTranslation=off  FrictionType=SmoothStickSlip  SenseFrictionalForceMagnitude=off  SenseNormalForceMagnitude=off  NormalForceType=SmoothSpringDamper  SenseNormalVelocity=off  SenseSeparationDistance=off  SenseTangentialVelocity=off  NormalTransitionRegionWidth=pkgGrndTransW  NormalTransitionRegionWidthUnits=m
  Spherical Solid : sm_lib/Body Elements/Spherical Solid  GraphicAmbientColor=[0.15 0.15 0.15 1.0]  BasedOnType=Density  CenterOfMass=[0 0 0]  CenterOfMassUnits=m  GraphicDiffuseColor=[0.5 0.5 0.5]  Density=1  DensityUnits=kg/m^3  DoExposeReferenceFrame=on  GraphicEmissiveColor=[0.0 0.0 0.0 1.0]  ExportEntireGeometry=on  SerializedExposedGeometries=<ExposedGeometries><ExposedGeometry><RawGeometryId>entire</RawGeometryId><ExposedGeometryId>G</ExposedGeometryId></ExposedGeometry></ExposedGeometries>  SerializedFrames=<Frames/>  MarkerShape=Sphere  MarkerSize=10  GraphicType=FromGeometry  InertiaType=CalculateFromGeometry  Mass=1  MassUnits=kg  MomentsOfInertia=[1 1 1]  MomentsOfInertiaUnits=kg*m^2  GraphicOpacity=1.0  ProductsOfInertia=[0 0 0]  ProductsOfInertiaUnits=kg*m^2  GraphicShininess=75  GraphicSpecularColor=[0.5 0.5 0.5 1.0]  SphereRadius=0.0025  SphereRadiusUnits=m  GraphicVisPropType=SimpleVisualProperties
  R : PMIOPort  Side=Right
  G : PMIOPort  Port=2  Side=Left
  connections:
  Spatial Contact Force/RConn1 -- G/RConn1
  Spherical Solid/RConn1 -- R/RConn1
  Spatial Contact Force/LConn1 -- Spherical Solid/LConn1

== system sm_quadcopter/Package Delivery Quadcopter/Package/Subsystem6 ==
  Spatial Contact Force : sm_lib/Forces and Torques/Spatial Contact Force  SenseContactBaseRotation=off  SenseContactBaseTranslation=off  CoefficientOfDynamicFriction=0.3  CoefficientOfStaticFriction=0.5  NormalDamping=pkgGrndDamp  NormalDampingUnits=N/(m/s)  SenseContactSignal=off  NormalStiffness=pkgGrndStiff  NormalStiffnessUnits=N/m  FrictionalCriticalVelocity=1e-2  FrictionalCriticalVelocityUnits=m/s  ZeroCrossDetectContactStartAndEnd=off  SenseContactFollowerRotation=off  SenseContactFollowerTranslation=off  FrictionType=SmoothStickSlip  SenseFrictionalForceMagnitude=off  SenseNormalForceMagnitude=off  NormalForceType=SmoothSpringDamper  SenseNormalVelocity=off  SenseSeparationDistance=off  SenseTangentialVelocity=off  NormalTransitionRegionWidth=pkgGrndTransW  NormalTransitionRegionWidthUnits=m
  Spherical Solid : sm_lib/Body Elements/Spherical Solid  GraphicAmbientColor=[0.15 0.15 0.15 1.0]  BasedOnType=Density  CenterOfMass=[0 0 0]  CenterOfMassUnits=m  GraphicDiffuseColor=[0.5 0.5 0.5]  Density=1  DensityUnits=kg/m^3  DoExposeReferenceFrame=on  GraphicEmissiveColor=[0.0 0.0 0.0 1.0]  ExportEntireGeometry=on  SerializedExposedGeometries=<ExposedGeometries><ExposedGeometry><RawGeometryId>entire</RawGeometryId><ExposedGeometryId>G</ExposedGeometryId></ExposedGeometry></ExposedGeometries>  SerializedFrames=<Frames/>  MarkerShape=Sphere  MarkerSize=10  GraphicType=FromGeometry  InertiaType=CalculateFromGeometry  Mass=1  MassUnits=kg  MomentsOfInertia=[1 1 1]  MomentsOfInertiaUnits=kg*m^2  GraphicOpacity=1.0  ProductsOfInertia=[0 0 0]  ProductsOfInertiaUnits=kg*m^2  GraphicShininess=75  GraphicSpecularColor=[0.5 0.5 0.5 1.0]  SphereRadius=0.0025  SphereRadiusUnits=m  GraphicVisPropType=SimpleVisualProperties
  R : PMIOPort  Side=Right
  G : PMIOPort  Port=2  Side=Left
  connections:
  Spatial Contact Force/LConn1 -- Spherical Solid/LConn1
  Spherical Solid/RConn1 -- R/RConn1
  Spatial Contact Force/RConn1 -- G/RConn1

== system sm_quadcopter/Package Delivery Quadcopter/Package/Subsystem7 ==
  Spatial Contact Force : sm_lib/Forces and Torques/Spatial Contact Force  SenseContactBaseRotation=off  SenseContactBaseTranslation=off  CoefficientOfDynamicFriction=0.3  CoefficientOfStaticFriction=0.5  NormalDamping=pkgGrndDamp  NormalDampingUnits=N/(m/s)  SenseContactSignal=off  NormalStiffness=pkgGrndStiff  NormalStiffnessUnits=N/m  FrictionalCriticalVelocity=1e-2  FrictionalCriticalVelocityUnits=m/s  ZeroCrossDetectContactStartAndEnd=off  SenseContactFollowerRotation=off  SenseContactFollowerTranslation=off  FrictionType=SmoothStickSlip  SenseFrictionalForceMagnitude=off  SenseNormalForceMagnitude=off  NormalForceType=SmoothSpringDamper  SenseNormalVelocity=off  SenseSeparationDistance=off  SenseTangentialVelocity=off  NormalTransitionRegionWidth=pkgGrndTransW  NormalTransitionRegionWidthUnits=m
  Spherical Solid : sm_lib/Body Elements/Spherical Solid  GraphicAmbientColor=[0.15 0.15 0.15 1.0]  BasedOnType=Density  CenterOfMass=[0 0 0]  CenterOfMassUnits=m  GraphicDiffuseColor=[0.5 0.5 0.5]  Density=1  DensityUnits=kg/m^3  DoExposeReferenceFrame=on  GraphicEmissiveColor=[0.0 0.0 0.0 1.0]  ExportEntireGeometry=on  SerializedExposedGeometries=<ExposedGeometries><ExposedGeometry><RawGeometryId>entire</RawGeometryId><ExposedGeometryId>G</ExposedGeometryId></ExposedGeometry></ExposedGeometries>  SerializedFrames=<Frames/>  MarkerShape=Sphere  MarkerSize=10  GraphicType=FromGeometry  InertiaType=CalculateFromGeometry  Mass=1  MassUnits=kg  MomentsOfInertia=[1 1 1]  MomentsOfInertiaUnits=kg*m^2  GraphicOpacity=1.0  ProductsOfInertia=[0 0 0]  ProductsOfInertiaUnits=kg*m^2  GraphicShininess=75  GraphicSpecularColor=[0.5 0.5 0.5 1.0]  SphereRadius=0.0025  SphereRadiusUnits=m  GraphicVisPropType=SimpleVisualProperties
  R : PMIOPort  Side=Right
  G : PMIOPort  Port=2  Side=Left
  connections:
  Spatial Contact Force/RConn1 -- G/RConn1
  Spherical Solid/RConn1 -- R/RConn1
  Spatial Contact Force/LConn1 -- Spherical Solid/LConn1

== matlab function sm_quadcopter/Trajectory Generation and Control/Position and Attitude Controller/Position Controller ==
  data: des_pos input; des_vel input; des_yaw input; pos input; vel input; pitch_des output; roll_des output; yaw_des output; attitude input; kp_position input; kd_position input
function [pitch_des,roll_des,yaw_des] = position_controller(des_pos,des_vel,des_yaw,pos,vel,attitude, kp_position, kd_position)
% This MATLAB function computes the desired roll, pitch and yaw angles to
% control the position of the quadcopter.

% Euler Angles
phi = attitude(1);
theta = attitude(2);
psi = attitude(3);

%% Obtain the desired state

% Direction Cosine Matrix
DCM = [cos(theta)*cos(psi)                                    cos(theta)*sin(psi)                          -sin(theta);
    -cos(phi)*sin(psi)+sin(phi)*sin(theta)*cos(psi) cos(phi)*cos(psi)+sin(phi)*sin(theta)*sin(psi) sin(phi)*cos(theta);
    sin(phi)*sin(psi)+cos(phi)*sin(theta)*cos(psi) -sin(phi)*cos(psi)+cos(phi)*sin(theta)*sin(psi) cos(phi)*cos(theta)];

% Desired Velocity
v_des = DCM*((des_vel - vel) + kp_position*(des_pos - pos));

% Desired Roll, Pitch and Yaw
pitch_des   = (1/(9.81))*(kd_position*v_des(1)); 
roll_des   = (-1/(9.81))*(kd_position*v_des(2)); 
yaw_des = des_yaw;
end

== matlab function sm_quadcopter/Package Delivery Quadcopter/Quadcopter Chassis/Quaternion to Euler Angles Conversion ==
  data: Quaternion input; roll output; pitch output; yaw output
function [roll,pitch,yaw] = quaternion_to_euler_angles_conversion(Quaternion)
% This MATLAB function converts the quaternions to the Euler Angles

w = Quaternion(1,1);
x = Quaternion(2,1);
y = Quaternion(3,1);
z = Quaternion(4,1);

% roll (x-axis rotation)
sinr_cosp = 2 * (w * x + y * z);
cosr_cosp = 1 - 2 * (x * x + y * y);
roll = atan2(sinr_cosp, cosr_cosp);

% pitch (y-axis rotation)
sinp = 2 * (w * y - z * x);
pitch = asin(sinp);

% yaw (z-axis rotation)
siny_cosp = 2 * (w * z + x * y);
cosy_cosp = 1 - 2 * (y * y + z * z);
yaw = atan2(siny_cosp, cosy_cosp);

end

== matlab function sm_quadcopter/Trajectory Generation and Control/Trajectory Generator ==
  settings: updateMethod=DISCRETE
  data: t input; pos_des output; vel_des output; yaw_des output; homePose input; timespot input; waypoints input; pos input
function [pos_des,vel_des,yaw_des]  = trajectory_generator(t,homePose,timespot,waypoints, pos)
% This MATLAB function is used to calculate the desired trajectory for the
% quadcopter.

persistent distance2waypoint waypointCounter px py pz;
persistent t0 tf X0 Y0 Z0 Xf Yf Zf vx0 vy0 vz0 vxf vyf vzf ax0 ay0 az0 axf ayf azf;

%% Calculate the desired trajectory from the home position to the first waypoint
if isempty(waypointCounter)
    waypointCounter   = 1;
    
    % Distance to the First Waypoint
    distance2waypoint = sqrt((homePose(1,1) - waypoints(1,1))^2 + (homePose(2,1) - waypoints(2,1))^2 + (homePose(3,1) - waypoints(3,1))^2);
    
    % Boundary Conditions
    
    % Time
    t0 = 0;
    tf = timespot(waypointCounter,1);
    
    % Position
    X0 = homePose(1,1);
    Y0 = homePose(2,1);
    Z0 = homePose(3,1);
    Xf = waypoints(1,1);
    Yf = waypoints(2,1);
    Zf = waypoints(3,1);
    
    % Velocity
    vx0 = 0;
    vy0 = 0;
    vz0 = 0;
    vxf = 0;
    vyf = 0;
    vzf = 0;
    
    % Acceleration
    ax0 = 0;
    ay0 = 0;
    az0 = 0;
    axf = 0;
    ayf = 0;
    azf = 0;
    
    A = [1 t0 t0^2 t0^3 t0^4 t0^5;...
        0 1 2*t0 3*t0^2 4*t0^3 5*t0^4;...
        0 0 2 6*t0 12*t0^2 20*t0^3;...
        1 tf tf^2 tf^3 tf^4 tf^5;...
        0 1 2*tf 3*tf^2 4*tf^3 5*tf^4;...
        0 0 2 6*tf 12*tf^2 20*tf^3];
    
    % Calculate the Trajectory Polynomials
    px = A\[X0 vx0 ax0 Xf vxf axf]';
    py = A\[Y0 vy0 ay0 Yf vyf ayf]';
    pz = A\[Z0 vz0 az0 Zf vzf azf]';
end

%% If the quadcopter is within the proximity of the Waypoint, compute the trajectory from the current waypoint to the next waypoint
if distance2waypoint <= 0.25
    
    % Update the waypointCounter
    waypointCounter = waypointCounter + 1;
    
    if waypointCounter <= length(waypoints)
        
        % Boundary Conditions
        
        % Time
        t0 = 0;
        tf = timespot(waypointCounter,1);
        
        % Position
        X0 = waypoints(1,waypointCounter-1);
        Y0 = waypoints(2,waypointCounter-1);
        Z0 = waypoints(3,waypointCounter-1);
        Xf = waypoints(1,waypointCounter);
        Yf = waypoints(2,waypointCounter);
        Zf = waypoints(3,waypointCounter);
        
        % Velocity
        vx0 = 0;
        vy0 = 0;
        vz0 = 0;
        vxf = 0;
        vyf = 0;
        vzf = 0;
        
        % Acceleration
        ax0 = 0;
        ay0 = 0;
        az0 = 0;
        axf = 0;
        ayf = 0;
        azf = 0;
        
        A = [1 t0 t0^2 t0^3 t0^4 t0^5;...
            0 1 2*t0 3*t0^2 4*t0^3 5*t0^4;...
            0 0 2 6*t0 12*t0^2 20*t0^3;...
            1 tf tf^2 tf^3 tf^4 tf^5;...
            0 1 2*tf 3*tf^2 4*tf^3 5*tf^4;...
            0 0 2 6*tf 12*tf^2 20*tf^3];
        
        % Calculate the Trajectory Polynomials
        px = A\[X0 vx0 ax0 Xf vxf axf]';
        py = A\[Y0 vy0 ay0 Yf vyf ayf]';
        pz = A\[Z0 vz0 az0 Zf vzf azf]';
        t0 = t;
    end
end

%% If the quadcopter has reached the target, then hover at the target location
if waypointCounter > length(waypoints)
    pos_des = waypoints(:,end);
    vel_des = [0;0;0];
else
    
    % Proceed to the next waypoint
    distance2waypoint = sqrt((pos(1,1) - waypoints(1,waypointCounter))^2 + (pos(2,1) - waypoints(2,waypointCounter))^2 + (pos(3,1) - waypoints(3,waypointCounter))^2);
    
    t_elapsed = t-t0;
    
    if t_elapsed < tf
        pos_des = [(px(6,1)*t_elapsed^5 + px(5,1)*t_elapsed^4 + px(4,1)*t_elapsed^3 + px(3,1)*t_elapsed^2 + px(2,1)*t_elapsed + px(1,1));...
            (py(6,1)*t_elapsed^5 + py(5,1)*t_elapsed^4 + py(4,1)*t_elapsed^3 + py(3,1)*t_elapsed^2 + py(2,1)*t_elapsed + py(1,1));...
            (pz(6,1)*t_elapsed^5 + pz(5,1)*t_elapsed^4 + pz(4,1)*t_elapsed^3 + pz(3,1)*t_elapsed^2 + pz(2,1)*t_elapsed + pz(1,1))];
        
        vel_des = [(5*px(6,1)*t_elapsed^4 + 4*px(5,1)*t_elapsed^3 + 3*px(4,1)*t_elapsed^2 + 2*px(3,1)*t_elapsed + px(2,1));...
            (5*py(6,1)*t_elapsed^4 + 4*py(5,1)*t_elapsed^3 + 3*py(4,1)*t_elapsed^2 + 2*py(3,1)*t_elapsed + py(2,1));...
            (5*pz(6,1)*t_elapsed^4 + 4*pz(5,1)*t_elapsed^3 + 3*pz(4,1)*t_elapsed^2 + 2*pz(3,1)*t_elapsed + pz(2,1))];
    else
        pos_des = [Xf;Yf;Zf];
        vel_des = [0;0;0];
    end
end

%% Desired Heading Angle
yaw_des = 0;
end

== matlab function sm_quadcopter/Package Delivery Quadcopter/Package Release Trigger ==
  settings: updateMethod=DISCRETE
  data: targetPos_X input; targetPos_Y input; targetPos_Z input; packagePos_X input; releaseTrigger output; packagePos_Y input; packagePos_Z input
function releaseTrigger = package_release_trigger(targetPos_X, targetPos_Y, targetPos_Z, packagePos_X, packagePos_Y, packagePos_Z)
% This MATLAB function sends a trigger signal to disengage the weld joint
% between the quadcopter and the package 

persistent releaseObj;

if sqrt((packagePos_X - targetPos_X)^2 + (packagePos_Y - targetPos_Y)^2 + (packagePos_Z - targetPos_Z)^2) < 0.3  && isempty(releaseObj)
    releaseTrigger = -1;
    releaseObj = 1;
elseif ~isempty(releaseObj)
    releaseTrigger = -1;
else
    releaseTrigger = 0;
end
end
